simulink model "H6bridge_single_phase_inverter"  (R2020b)
settings: Solver=FixedStepDiscrete  StartTime=0.0  StopTime=2  FixedStep=5e-7  RelTol=1e-3
libraries: powerlib x17, pid_lib x1, simulink x1
settings Model: Creator=gc45  LastModifiedBy=gc45
settings DataIOCC: ReturnWorkspaceOutputs=off

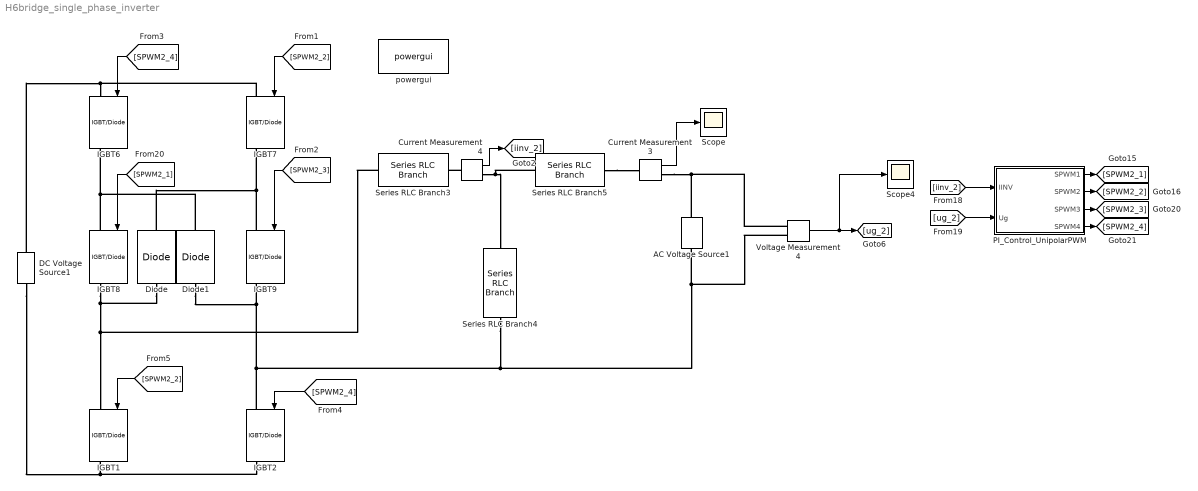
== system H6bridge_single_phase_inverter ==
  AC Voltage Source1 : powerlib/Electrical Sources/AC Voltage Source  Amplitude=311  Phase=0  Frequency=50  SampleTime=0  Measurements=None  BusType=swing  Pref=10e3  Qref=0  Qmin=-inf  Qmax=+inf
  Current Measurement3 : powerlib/Measurements/Current Measurement  PhasorSimulation=off  OutputType=Complex  PSBequivalent=0
  Current Measurement4 : powerlib/Measurements/Current Measurement  PhasorSimulation=off  OutputType=Complex  PSBequivalent=0
  DC Voltage Source1 : powerlib/Electrical Sources/DC Voltage Source  Amplitude=400  Measurements=None
  Diode : powerlib/Power Electronics/Diode  Ron=0.001  Lon=0  Vf=0.8  IC=0  UseSnubber=0  Rs=500  Cs=250e-9  Measurements=off
  Diode1 : powerlib/Power Electronics/Diode  Ron=0.001  Lon=0  Vf=0.8  IC=0  UseSnubber=0  Rs=500  Cs=250e-9  Measurements=off
  IGBT{1..2,6..9} (6 alike) : powerlib/Power Electronics/IGBT//Diode  Ron=1e-3  Rs=1e5  Cs=inf  Measurements=on
  PI_Control_UnipolarPWM : Subsystem
  Scope : Scope
  Scope4 : Scope
  Series RLC Branch3 : powerlib/Elements/Series RLC Branch  LConnTagsString=__new0  RConnTagsString=__new0  BranchType=L  Resistance=0.01  Inductance=4.06e-3  SetiL0=off  InitialCurrent=0  Capacitance=1e-6  Setx0=off  InitialVoltage=0  Measurements=None
  Series RLC Branch4 : powerlib/Elements/Series RLC Branch  LConnTagsString=__new0  RConnTagsString=__new0  BranchType=C  Resistance=0.01  Inductance=20e-3  SetiL0=off  InitialCurrent=0  Capacitance=6e-6  Setx0=off  InitialVoltage=0  Measurements=None
  Series RLC Branch5 : powerlib/Elements/Series RLC Branch  LConnTagsString=__new0  RConnTagsString=__new0  BranchType=L  Resistance=0.01  Inductance=4.35e-3  SetiL0=off  InitialCurrent=0  Capacitance=1e-6  Setx0=off  InitialVoltage=0  Measurements=None
  Voltage Measurement4 : powerlib/Measurements/Voltage Measurement  PhasorSimulation=off  OutputType=Complex  PSBequivalent=0
  powergui : powerlib/powergui  Priority=1  SimulationMode=Discrete  SampleTime=1e-6  frequency=60  Iterations=50  frequencyindice=50  Pbase=100e6  ErrMax=1e-4  UnitsV=kV  UnitsW=MW  buscounter=0  FunctionMessages=off  echomessages=off  EnableUseOfTLC=off  CurrentSourceSwitches=off  DisableSnubberDevices=off  DisableRonSwitches=off  DisableVfSwitches=off  DisplayEquations=off  AutomaticDiscreteSolvers=off  SolverType=Tustin/Backward Euler (TBE)  Interpol=off  ExternalGateDelay=off  methode=off  Ts=100  x0status=blocks  SPID=on  SwTol=0  HookPort=off  NonlinearTolerance=1e-4  nMaxIteration=100  ContinueOnMaxIteration=off  RestoreLinks=warning  ResistiveCurrentMeasurement=off  Frange=[0:2:500]  Ylog=off  Xlog=on  ShowGrid=off  save=off  variable=ZData  structure=ig  ZoomFFT=off  StartTime=1  cycles=40  DisplayStyle=2  fundamental=50  FreqAxis=off  MaxFrequency=1000  frequencyindicesteady=1  RmsSteady=1  display=off
  wires:
  [iinv_2] -> PI_Control_UnipolarPWM/1(IINV)
  Voltage Measurement4/1 -> Scope4/1, [ug_2]
  [ug_2] -> PI_Control_UnipolarPWM/2(Ug)
  PI_Control_UnipolarPWM/4(SPWM4) -> [SPWM2_4]
  PI_Control_UnipolarPWM/1(SPWM1) -> [SPWM2_1]
  PI_Control_UnipolarPWM/3(SPWM3) -> [SPWM2_3]
  PI_Control_UnipolarPWM/2(SPWM2) -> [SPWM2_2]
  [SPWM2_3] -> IGBT9/1
  [SPWM2_4] -> IGBT6/1
  Current Measurement4/1 -> [iinv_2]
  Current Measurement3/1 -> Scope/1
  [SPWM2_2] -> IGBT7/1
  [SPWM2_1] -> IGBT8/1
  [SPWM2_4] -> IGBT2/1
  [SPWM2_2] -> IGBT1/1
  connections:
  AC Voltage Source1/RConn1 -- Voltage Measurement4/LConn1 -- Current Measurement3/RConn1
  Current Measurement4/RConn1 -- Series RLC Branch4/LConn1 -- Series RLC Branch5/LConn1
  DC Voltage Source1/RConn1 -- IGBT7/LConn1 -- IGBT6/LConn1
  Series RLC Branch5/RConn1 -- Current Measurement3/LConn1
  Current Measurement4/LConn1 -- Series RLC Branch3/RConn1
  IGBT8/RConn1 -- Diode/LConn1 -- Series RLC Branch3/LConn1 -- IGBT1/LConn1
  Voltage Measurement4/LConn2 -- Series RLC Branch4/RConn1 -- IGBT2/LConn1 -- Diode1/LConn1 -- IGBT9/RConn1 -- AC Voltage Source1/LConn1
  DC Voltage Source1/LConn1 -- IGBT2/RConn1 -- IGBT1/RConn1
  IGBT9/LConn1 -- Diode/RConn1 -- IGBT7/RConn1
  IGBT8/LConn1 -- Diode1/RConn1 -- IGBT6/RConn1

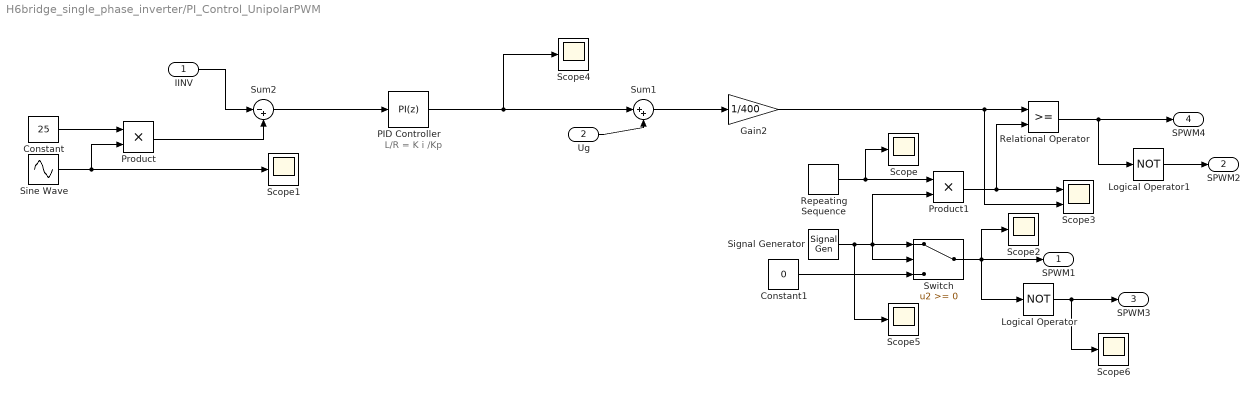
== system H6bridge_single_phase_inverter/PI_Control_UnipolarPWM ==
  note: L/R = K i /Kp
  IINV : Inport
  Ug : Inport  Port=2
  Constant : Constant  Value=25
  Constant1 : Constant  Value=0
  Gain2 : Gain  Gain=1/400
  Logical Operator : Logic  Operator=NOT  AllPortsSameDT=off  OutDataTypeStr=boolean
  Logical Operator1 : Logic  Operator=NOT  AllPortsSameDT=off  OutDataTypeStr=boolean
  PID Controller : pid_lib/PID Controller  Controller=PI  Form=Parallel  TimeDomain=Discrete-time  UseExternalTs=off  SampleTime=-1  IntegratorMethod=Forward Euler  FilterMethod=Forward Euler  ControllerParametersSource=internal  P=5  I=500  D=0  UseFilter=on  N=100  TunerSelectOption=Transfer Function Based (PID Tuner App)  InitialConditionSource=internal  InitialConditionForIntegrator=0  InitialConditionForFilter=0  DifferentiatorICPrevScaledInput=0  ExternalReset=none  TrackingMode=off  Kt=1  LimitOutput=off  SatLimitsSource=internal  UpperSaturationLimit=inf  LowerSaturationLimit=-inf  LinearizeAsGain=on  AntiWindupMode=none  Kb=1  POutMin=[]  POutMax=[]  IOutMin=[]  IOutMax=[]  DOutMin=[]  DOutMax=[]  NOutMin=[]  NOutMax=[]  SumOutMin=[]  SumOutMax=[]  SaturationOutMin=[]  SaturationOutMax=[]  PParamMin=[]  PParamMax=[]  IParamMin=[]  IParamMax=[]  DParamMin=[]  DParamMax=[]  NParamMin=[]  NParamMax=[]  KbParamMin=[]  KbParamMax=[]  KtParamMin=[]  KtParamMax=[]  KbOutMin=[]  KbOutMax=[]  KtOutMin=[]  KtOutMax=[]  IntegratorOutMin=[]  IntegratorOutMax=[]  FilterOutMin=[]  FilterOutMax=[]  SumI1OutMin=[]  SumI1OutMax=[]  SumI2OutMin=[]  SumI2OutMax=[]  SumI3OutMin=[]  SumI3OutMax=[]  SumI4OutMin=[]  SumI4OutMax=[]  SumDOutMin=[]  SumDOutMax=[]  DifferentiatorOutMin=[]  DifferentiatorOutMax=[]  FilterDiffOutCoefMin=[]  FilterDiffOutCoefMax=[]  ReciprocalOutMin=[]  ReciprocalOutMax=[]  SumDenOutMin=[]  SumDenOutMax=[]  SumNumOutMin=[]  SumNumOutMax=[]  DivideOutMin=[]  DivideOutMax=[]  UdiffTsProdOutMin=[]  UdiffTsProdOutMax=[]  NTsProdOutMin=[]  NTsProdOutMax=[]  UintegralTsProdOutMin=[]  UintegralTsProdOutMax=[]  UngainTsProdOutMin=[]  UngainTsProdOutMax=[]  IntegratorContinuousStateAttributes=''  IntegratorStateMustResolveToSignalObject=off  IntegratorRTWStateStorageClass=Auto  FilterContinuousStateAttributes=''  FilterStateMustResolveToSignalObject=off  FilterRTWStateStorageClass=Auto  ParallelPVariant=InternalParameters  IdealPVariant=Disabled  IVariant=InternalParameters  DVariant=Disabled  IntegratorVariant=Discrete  SatVariant=Disabled  AWVariant=Passthrough  PCopyVariant=Disabled  TRVariant=Disabled  FdbkBlocksVariant=Forward  IdealPFdbkVariant=Disabled  SatFdbkVariant=Disabled  DerivativeFilterVariant=Disabled  NVariant=Disabled  NCopyVariant=Disabled_SignalSpec  FilterICVariant=Disabled  IntegratorICVariant=InternalICs  ExternalResetVariant=Disabled  TRSumVariant=Passthrough  SumFdbkVariant=Disabled  SumVariant=Sum_PI  TsampFilterVariant=InternalTs  TsampNgainVariant=Passthrough  TsampIntegralVariant=Passthrough  ExternalSaturationOutDataTypeStr=Inherit: Same as second input
  Product : Product
  Product1 : Product
  Relational Operator : RelationalOperator  OutDataTypeStr=boolean  RndMeth=Simplest
  Repeating Sequence : simulink/Sources/Repeating Sequence  rep_seq_t=[0 1/20000 1/10000]  rep_seq_y=[0 1 0]
  Scope{,1..2,4..6} (6 alike) : Scope
  Scope3 : Scope  NumInputPorts=2
  Signal Generator : SignalGenerator  WaveForm=square  Amplitude=-1  Frequency=50*2*pi  Units=rad/sec
  Sine Wave : Sin  Frequency=100*pi  SampleTime=1e-6
  Sum1 : Sum  Inputs=|++
  Sum2 : Sum  Inputs=|-+
  Switch : Switch
  SPWM1 : Outport
  SPWM2 : Outport  Port=2
  SPWM3 : Outport  Port=3
  SPWM4 : Outport  Port=4
  wires:
  Sum2/1 -> PID Controller/1
  Product/1 -> Sum2/2
  IINV/1 -> Sum2/1
  Constant/1 -> Product/1
  Sine Wave/1 -> Scope1/1, Product/2
  Ug/1 -> Sum1/2
  Signal Generator/1 -> Scope5/1, Product1/2, Switch/2, Switch/1
  Repeating Sequence/1 -> Scope/1, Product1/1
  Product1/1 -> Relational Operator/2, Scope3/1
  Constant1/1 -> Switch/3
  Switch/1 -> SPWM1/1, Logical Operator/1, Scope2/1
  PID Controller/1 -> Scope4/1, Sum1/1
  Sum1/1 -> Gain2/1
  Gain2/1 -> Scope3/2, Relational Operator/1
  Relational Operator/1 -> Logical Operator1/1, SPWM4/1
  Logical Operator1/1 -> SPWM2/1
  Logical Operator/1 -> SPWM3/1, Scope6/1
